simulink model "Starfighter_6DoF_runsim_waypoint"  (R2013b)
settings: Solver=ode4  StartTime=0.0  StopTime=1  FixedStep=.01  MaxStep=.004  RelTol=1e-5
values from neighbouring files (symbols this model uses):
  a = 967.78    [LocusTrans.m]    (also in runsim_Starfighter_6DoF_Waypoint.m)
  ac = [0 0 0]    [LocusTrans.m]    (also in runsim_Starfighter_6DoF_Waypoint.m)
  b = 21.9    [LocusTrans.m]    (also in runsim_Starfighter_6DoF_Waypoint.m)
  cbar = 9.6    [LocusTrans.m]    (also in runsim_Starfighter_6DoF_Waypoint.m)
  cda = 0.384    [LocusTrans.m]    (also in runsim_Starfighter_6DoF_Waypoint.m)
  cdde = 0    [LocusTrans.m]    (also in runsim_Starfighter_6DoF_Waypoint.m)
  cdo = 0.048    [LocusTrans.m]    (also in runsim_Starfighter_6DoF_Waypoint.m)
  cg = [0 0 0]    [LocusTrans.m]    (also in runsim_Starfighter_6DoF_Waypoint.m)
  cla = 2.005    [LocusTrans.m]    (also in runsim_Starfighter_6DoF_Waypoint.m)
  cladot = 0.82    [LocusTrans.m]    (also in runsim_Starfighter_6DoF_Waypoint.m)
  clb = -0.093    [LocusTrans.m]    (also in runsim_Starfighter_6DoF_Waypoint.m)
  clda = 0.0173    [LocusTrans.m]    (also in runsim_Starfighter_6DoF_Waypoint.m)
  clde = 0.523    [LocusTrans.m]    (also in runsim_Starfighter_6DoF_Waypoint.m)
  cldr = 0.0079    [LocusTrans.m]    (also in runsim_Starfighter_6DoF_Waypoint.m)
  clo = 0.122    [LocusTrans.m]    (also in runsim_Starfighter_6DoF_Waypoint.m)
  clp = -0.272    [LocusTrans.m]    (also in runsim_Starfighter_6DoF_Waypoint.m)
  clq = 1.9    [LocusTrans.m]    (also in runsim_Starfighter_6DoF_Waypoint.m)
  clr = 0.154    [LocusTrans.m]    (also in runsim_Starfighter_6DoF_Waypoint.m)
  cma = -1.308    [LocusTrans.m]    (also in runsim_Starfighter_6DoF_Waypoint.m)
  cmadot = -2.05    [LocusTrans.m]    (also in runsim_Starfighter_6DoF_Waypoint.m)
  cmde = -1.31    [LocusTrans.m]    (also in runsim_Starfighter_6DoF_Waypoint.m)
  cmo = -0.028    [LocusTrans.m]    (also in runsim_Starfighter_6DoF_Waypoint.m)
  cmq = -4.83    [LocusTrans.m]    (also in runsim_Starfighter_6DoF_Waypoint.m)
  cnb = 0.242    [LocusTrans.m]    (also in runsim_Starfighter_6DoF_Waypoint.m)
  cnda = -0.0025    [LocusTrans.m]    (also in runsim_Starfighter_6DoF_Waypoint.m)
  cndr = -0.0435    [LocusTrans.m]    (also in runsim_Starfighter_6DoF_Waypoint.m)
  cnp = -0.093    [LocusTrans.m]    (also in runsim_Starfighter_6DoF_Waypoint.m)
  cnr = -0.649    [LocusTrans.m]    (also in runsim_Starfighter_6DoF_Waypoint.m)
  cyb = -1.045    [LocusTrans.m]    (also in runsim_Starfighter_6DoF_Waypoint.m)
  cyda = 0    [LocusTrans.m]    (also in runsim_Starfighter_6DoF_Waypoint.m)
  cydr = 0.087    [LocusTrans.m]    (also in runsim_Starfighter_6DoF_Waypoint.m)
  cyp = 0    [LocusTrans.m]    (also in runsim_Starfighter_6DoF_Waypoint.m)
  cyr = 0    [LocusTrans.m]    (also in runsim_Starfighter_6DoF_Waypoint.m)
  de0 = -4.1938979*pi/180    (= -0.0731973268475)    [LocusTrans.m]    (also in runsim_Starfighter_6DoF_Waypoint.m)
  dT0 = 5795.5876705721688901230688059874    (= 5795.58767057)    [LocusTrans.m]    (also in runsim_Starfighter_6DoF_Waypoint.m = 0.4868)
  eng = [0 0 0]    [LocusTrans.m]    (also in runsim_Starfighter_6DoF_Waypoint.m)
  inialt = 55000    [runsim_Starfighter_6DoF_Waypoint.m]
  initalt = 0    [LocusTrans.m]    (also in runsim_Starfighter_6DoF_Waypoint.m = 55000)
  initeast = 0    [LocusTrans.m]    (also in runsim_Starfighter_6DoF_Waypoint.m)
  initnorth = 0    [LocusTrans.m]    (also in runsim_Starfighter_6DoF_Waypoint.m)
  initp = p0    (= 0)    [LocusTrans.m]    (also in runsim_Starfighter_6DoF_Waypoint.m)
  initpitch = theta0    (= 0.0519025210107)    [LocusTrans.m]    (also in runsim_Starfighter_6DoF_Waypoint.m)
  initq = q0    (= 0)    [LocusTrans.m]    (also in runsim_Starfighter_6DoF_Waypoint.m)
  initr = r0    (= 0)    [LocusTrans.m]    (also in runsim_Starfighter_6DoF_Waypoint.m)
  initroll = phi0    (= 0)    [LocusTrans.m]    (also in runsim_Starfighter_6DoF_Waypoint.m)
  initu = u0    [LocusTrans.m]    (also in runsim_Starfighter_6DoF_Waypoint.m)
  initv = v0    [LocusTrans.m]    (also in runsim_Starfighter_6DoF_Waypoint.m)
  initw = w0    [LocusTrans.m]    (also in runsim_Starfighter_6DoF_Waypoint.m)
  inityaw = 0.0    (= 0)    [LocusTrans.m]    (also in runsim_Starfighter_6DoF_Waypoint.m)
  Ix = 3600    [LocusTrans.m]    (also in runsim_Starfighter_6DoF_Waypoint.m)
  Ixz = 0    [LocusTrans.m]    (also in runsim_Starfighter_6DoF_Waypoint.m)
  Iy = 59000    [LocusTrans.m]    (also in runsim_Starfighter_6DoF_Waypoint.m)
  Iz = 60000    [LocusTrans.m]    (also in runsim_Starfighter_6DoF_Waypoint.m)
  K_phi = 10    [runsim_Starfighter_6DoF_Waypoint.m]
  rho = .002378*(1-.0000068756*     h)^4.2561    (= 0.000314842619782)    [LocusTrans.m]    (also in runsim_Starfighter_6DoF_Waypoint.m)
  sw = 196    [LocusTrans.m]    (also in runsim_Starfighter_6DoF_Waypoint.m)
  T_max = 11905    [runsim_Starfighter_6DoF_Waypoint.m]
  u0 = Vt0*cos(alpha0)*cos(beta0)    [LocusTrans.m]    (also in runsim_Starfighter_6DoF_Waypoint.m)
  Vt0 = 1742    [Control.m]    (also in LocusTrans.m; runsim_Starfighter_6DoF_Waypoint.m)
  weight = 16300    [runsim_Starfighter_6DoF_Waypoint.m]
  Xw = (1/u0)*Xa    [LocusTrans.m]    (also in runsim_Starfighter_6DoF_Waypoint.m = 2*[52*Vt0, 104*Vt0, 104*Vt0, 52*Vt0, 0])
libraries: simulink x6, dspswit3 x1
(part 1 of 2)
settings Model: ExtModeAutoUpdateStatusClock=off  Creator=andersop  LastModifiedBy=mittalk1
settings SolverCC: InitialStep=.004
settings DataIOCC: SignalLoggingSaveFormat=ModelDataLogs  SaveState=on  SignalLoggingName=sigsOut
settings OptimizationCC: ExpressionDepthLimit=2147483647  InitFltsAndDblsToZero=on
settings DebuggingCC: SaveWithParameterizedLinksMsg=none  SignalResolutionControl=TryResolveAllWithWarning  SolverPrmCheckMsg=none  MultiTaskDSMMsg=warning  MultiTaskCondExecSysMsg=none  FcnCallInpInsideContextMsg=UseLocalSettings  StateNameClashWarn=warning
settings HardwareCC: TargetUnknown=on
settings RTWCC: IncludeERTFirstTime=on
settings GRTTargetCC: TargetFcnLib=ansi_tfl_tmw.mat  ModelReferenceCompliant=off  CombineOutputUpdateFcns=off  MatFileLogging=off  GRTInterface=on

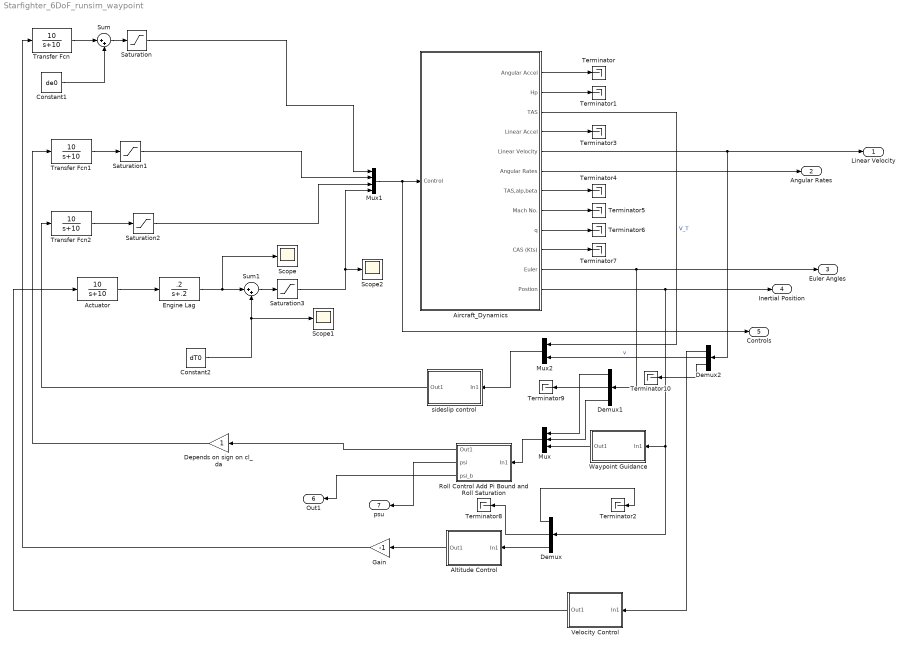
== system Starfighter_6DoF_runsim_waypoint ==
  Actuator : TransferFcn  Numerator=[10]  Denominator=[1 10]
  Aircraft_Dynamics : Subsystem
  Altitude Control : Subsystem
  Constant1 : Constant  Value=de0
  Constant2 : Constant  Value=dT0
  Demux : Demux  Outputs=3
  Demux1 : Demux  Outputs=3
  Demux2 : Demux  Outputs=3
  Depends on sign on cl_da : Gain
  Engine Lag : TransferFcn  Numerator=[.2]  Denominator=[1 .2]
  Gain : Gain  Gain=-1
  Mux : Mux  Inputs=3
  Mux1 : Mux
  Mux2 : Mux  Inputs=2
  Roll Control Add Pi Bound and Roll Saturation : Subsystem
  Saturation : Saturate  UpperLimit=30*pi/180  LowerLimit=-30*pi/180
  Saturation1 : Saturate  UpperLimit=40*pi/180  LowerLimit=-40*pi/180
  Saturation2 : Saturate  UpperLimit=30*pi/180  LowerLimit=-30*pi/180
  Saturation3 : Saturate  UpperLimit=1  LowerLimit=0
  Scope : Scope
      settings: YMin=0  YMax=0.025
  Scope1 : Scope
      settings: YMin=0.4868  YMax=0.4868
  Scope2 : Scope
      settings: YMin=0.485  YMax=0.5125  SaveName=ScopeData2
  Sum : Sum  Inputs=|++
  Sum1 : Sum  Inputs=|++
  Terminator{,1..10} (11 alike) : Terminator
  Transfer Fcn : TransferFcn  Numerator=[10]  Denominator=[1 10]
  Transfer Fcn1 : TransferFcn  Numerator=[10]  Denominator=[1 10]
  Transfer Fcn2 : TransferFcn  Numerator=[10]  Denominator=[1 10]
  Velocity Control : Subsystem
  Waypoint Guidance : Subsystem
  sideslip control : Subsystem
  Linear Velocity : Outport
  Angular Rates : Outport  Port=2
  Euler Angles : Outport  Port=3
  Inertial Position : Outport  Port=4
  Controls : Outport  Port=5
  Out1 : Outport  Port=6
  psu : Outport  Port=7
  wires:
  Aircraft_Dynamics/11(Euler) -> Demux1/1, Euler Angles/1
  Saturation3/1 -> Scope2/1, Mux1/4
  Mux1/1 -> Aircraft_Dynamics/1(Control), Controls/1
  Saturation/1 -> Mux1/1
  Aircraft_Dynamics/6(Angular Rates) -> Angular Rates/1
  Aircraft_Dynamics/5(Linear Velocity) -> Demux2/1, Linear Velocity/1
  Saturation2/1 -> Mux1/3
  Saturation1/1 -> Mux1/2
  Aircraft_Dynamics/1(Angular Accel) -> Terminator/1
  Aircraft_Dynamics/2(Hp) -> Terminator1/1
  Aircraft_Dynamics/3(TAS) -> Mux2/1  "V_T"
  Aircraft_Dynamics/4(Linear Accel) -> Terminator3/1
  Aircraft_Dynamics/7(TAS,alp,beta) -> Terminator4/1
  Aircraft_Dynamics/8(Mach No.) -> Terminator5/1
  Aircraft_Dynamics/10(CAS (Kts)) -> Terminator7/1
  Aircraft_Dynamics/9(q) -> Terminator6/1
  Sum/1 -> Saturation/1
  Constant1/1 -> Sum/2
  Transfer Fcn/1 -> Sum/1
  Transfer Fcn1/1 -> Saturation1/1
  Aircraft_Dynamics/12(Postion) -> Demux/1, Waypoint Guidance/1(In1), Inertial Position/1
  Waypoint Guidance/1(Out1) -> Mux/3
  Demux1/1 -> Mux/1
  Demux1/3 -> Mux/2
  Mux/1 -> Roll Control Add Pi Bound and Roll Saturation/1(In1)
  Depends on sign on cl_da/1 -> Transfer Fcn1/1
  Gain/1 -> Transfer Fcn/1
  Demux/3 -> Altitude Control/1(In1)
  Altitude Control/1(Out1) -> Gain/1
  Demux2/2 -> Mux2/2  "v"
  Transfer Fcn2/1 -> Saturation2/1
  sideslip control/1(Out1) -> Transfer Fcn2/1
  Demux/1 -> Terminator2/1
  Demux/2 -> Terminator8/1
  Demux1/2 -> Terminator9/1
  Demux2/1 -> Velocity Control/1(In1)
  Constant2/1 -> Scope1/1, Sum1/2
  Engine Lag/1 -> Scope/1, Sum1/1
  Actuator/1 -> Engine Lag/1
  Sum1/1 -> Saturation3/1
  Velocity Control/1(Out1) -> Actuator/1
  Demux2/3 -> Terminator10/1
  Roll Control Add Pi Bound and Roll Saturation/2(psi) -> psu/1
  Roll Control Add Pi Bound and Roll Saturation/3(psi_b) -> Out1/1
  Mux2/1 -> sideslip control/1(In1)
  Roll Control Add Pi Bound and Roll Saturation/1(Out1) -> Depends on sign on cl_da/1

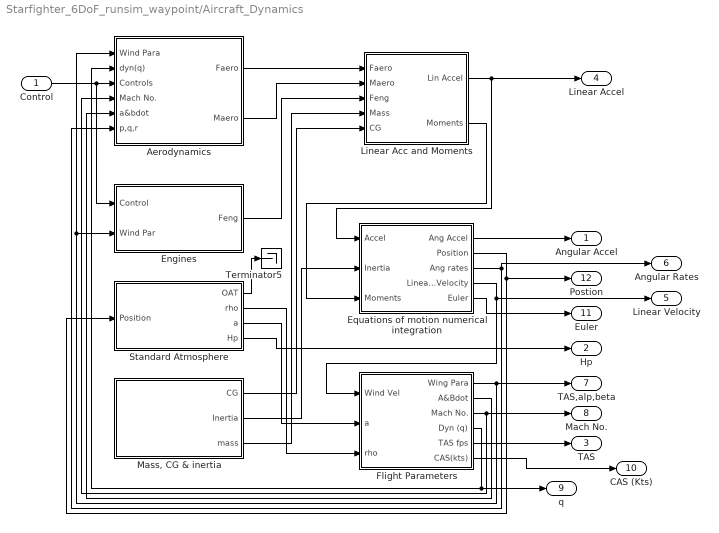
== system Starfighter_6DoF_runsim_waypoint/Aircraft_Dynamics ==
  Control : Inport
  Aerodynamics : Subsystem
  Engines : Subsystem
  "Equations of motion numerical integration " : Subsystem
  Flight Parameters : Subsystem
  Linear Acc and Moments : Subsystem
  "Mass, CG & inertia" : Subsystem
  Standard Atmosphere : Subsystem
  Terminator5 : Terminator
  Angular Accel : Outport
  Hp : Outport  Port=2
  TAS : Outport  Port=3
  Linear Accel : Outport  Port=4
  Linear Velocity : Outport  Port=5
  Angular Rates : Outport  Port=6
  TAS,alp,beta : Outport  Port=7
  Mach No. : Outport  Port=8
  q : Outport  Port=9
  CAS (Kts) : Outport  Port=10
  Euler : Outport  Port=11
  Postion : Outport  Port=12
  wires:
  Aerodynamics/1(Faero) -> Linear Acc and Moments/1(Faero)
  Aerodynamics/2(Maero) -> Linear Acc and Moments/2(Maero)
  Control/1 -> Aerodynamics/3(Controls), Engines/1(Control)
  Engines/1(Feng) -> Linear Acc and Moments/3(Feng)
  "Mass, CG & inertia"/1(CG) -> Linear Acc and Moments/5(CG)
  "Mass, CG & inertia"/2(Inertia) -> "Equations of motion numerical integration "/2(Inertia)
  Linear Acc and Moments/1(Lin Accel) -> "Equations of motion numerical integration "/1(Accel), Linear Accel/1
  Linear Acc and Moments/2(Moments) -> "Equations of motion numerical integration "/3(Moments)
  "Equations of motion numerical integration "/3(Ang rates) -> Aerodynamics/6(p,q,r), Angular Rates/1
  "Equations of motion numerical integration "/4(Linear Velocity) -> Flight Parameters/1(Wind Vel), Linear Velocity/1
  Flight Parameters/1(Wing Para) -> TAS,alp,beta/1, Aerodynamics/1(Wind Para), Engines/2(Wind Par)
  Flight Parameters/4(Dyn (q)) -> Aerodynamics/2(dyn(q)), q/1
  Flight Parameters/3(Mach No.) -> Mach No./1, Aerodynamics/4(Mach No.)
  Flight Parameters/2(A&Bdot) -> Aerodynamics/5(a&bdot)
  "Equations of motion numerical integration "/2(Position) -> Postion/1, Standard Atmosphere/1(Position)
  "Equations of motion numerical integration "/1(Ang Accel) -> Angular Accel/1
  Standard Atmosphere/4(Hp) -> Hp/1
  Flight Parameters/5(TAS fps) -> TAS/1
  Flight Parameters/6(CAS(kts)) -> CAS (Kts)/1
  "Equations of motion numerical integration "/5(Euler) -> Euler/1
  Standard Atmosphere/3(a) -> Flight Parameters/2(a)
  Standard Atmosphere/2(rho) -> Flight Parameters/3(rho)
  "Mass, CG & inertia"/3(mass) -> Linear Acc and Moments/4(Mass)
  Standard Atmosphere/1(OAT) -> Terminator5/1

== system Starfighter_6DoF_runsim_waypoint/Altitude Control ==
  In1 : Inport
  Altitude PID Controller : simulink/Continuous/PID Controller  Controller=PID  TimeDomain=Continuous-time  SampleTime=1  IntegratorMethod=Forward Euler  FilterMethod=Forward Euler  Form=Parallel  P=5.28484698542776e-05  I=1.87875420337088e-07  D=0.00194166371372168  N=0.684337429388764  InitialConditionSource=internal  InitialConditionForIntegrator=0  InitialConditionForFilter=0  ExternalReset=none  LimitOutput=off  UpperSaturationLimit=inf  LowerSaturationLimit=-inf  LinearizeAsGain=on  AntiWindupMode=none  Kb=1  TrackingMode=off  Kt=1  PParamMin=[]  PParamMax=[]  IParamMin=[]  IParamMax=[]  DParamMin=[]  DParamMax=[]  NParamMin=[]  NParamMax=[]  KbParamMin=[]  KbParamMax=[]  KtParamMin=[]  KtParamMax=[]  POutMin=[]  POutMax=[]  IOutMin=[]  IOutMax=[]  DOutMin=[]  DOutMax=[]  NOutMin=[]  NOutMax=[]  KbOutMin=[]  KbOutMax=[]  KtOutMin=[]  KtOutMax=[]  IntegratorOutMin=[]  IntegratorOutMax=[]  FilterOutMin=[]  FilterOutMax=[]  SumOutMin=[]  SumOutMax=[]  SumI1OutMin=[]  SumI1OutMax=[]  SumI2OutMin=[]  SumI2OutMax=[]  SumI3OutMin=[]  SumI3OutMax=[]  SumDOutMin=[]  SumDOutMax=[]  SaturationOutMin=[]  SaturationOutMax=[]  IntegratorContinuousStateAttributes=''  IntegratorStateMustResolveToSignalObject=off  IntegratorRTWStateStorageClass=Auto  FilterContinuousStateAttributes=''  FilterStateMustResolveToSignalObject=off  FilterRTWStateStorageClass=Auto
  Constant : Constant  Value=inialt
  Sum1 : Sum  Inputs=|-+
  Out1 : Outport
  wires:
  Sum1/1 -> Altitude PID Controller/1
  In1/1 -> Sum1/1
  Altitude PID Controller/1 -> Out1/1
  Constant/1 -> Sum1/2

== system Starfighter_6DoF_runsim_waypoint/Roll Control Add Pi Bound and Roll Saturation ==
  In1 : Inport
  Demux : Demux  Outputs=3
  Gain : Gain  Gain=K_phi
  PID Controller : simulink/Continuous/PID Controller  Controller=PID  TimeDomain=Continuous-time  SampleTime=1  IntegratorMethod=Forward Euler  FilterMethod=Forward Euler  Form=Parallel  P=0.0237928230779275  I=0.000453455739705604  D=0.0522613184684565  N=1.14124341327547  InitialConditionSource=internal  InitialConditionForIntegrator=0  InitialConditionForFilter=0  ExternalReset=none  LimitOutput=off  UpperSaturationLimit=inf  LowerSaturationLimit=-inf  LinearizeAsGain=on  AntiWindupMode=none  Kb=1  TrackingMode=off  Kt=1  PParamMin=[]  PParamMax=[]  IParamMin=[]  IParamMax=[]  DParamMin=[]  DParamMax=[]  NParamMin=[]  NParamMax=[]  KbParamMin=[]  KbParamMax=[]  KtParamMin=[]  KtParamMax=[]  POutMin=[]  POutMax=[]  IOutMin=[]  IOutMax=[]  DOutMin=[]  DOutMax=[]  NOutMin=[]  NOutMax=[]  KbOutMin=[]  KbOutMax=[]  KtOutMin=[]  KtOutMax=[]  IntegratorOutMin=[]  IntegratorOutMax=[]  FilterOutMin=[]  FilterOutMax=[]  SumOutMin=[]  SumOutMax=[]  SumI1OutMin=[]  SumI1OutMax=[]  SumI2OutMin=[]  SumI2OutMax=[]  SumI3OutMin=[]  SumI3OutMax=[]  SumDOutMin=[]  SumDOutMax=[]  SaturationOutMin=[]  SaturationOutMax=[]  IntegratorContinuousStateAttributes=''  IntegratorStateMustResolveToSignalObject=off  IntegratorRTWStateStorageClass=Auto  FilterContinuousStateAttributes=''  FilterStateMustResolveToSignalObject=off  FilterRTWStateStorageClass=Auto
  Saturation : Saturate  UpperLimit=40*(pi/180)  LowerLimit=-40*(pi/180)
  Sum : Sum  Inputs=|-+
  Sum1 : Sum  Inputs=|-+
  pi Bound1 : Subsystem  mask(pi bound){}
      mask help: Bounds the input angle to [-pi, pi]. When -pi bound is exceeded the output wraps back to pi; when the pi bound is exceeded the output wraps back to -pi.
      mask Help:
      | Bounds the input angle to [-pi, pi]. When -pi bound is exceeded the output wraps back to pi; when the pi bound is exceeded the output wraps back to -pi.
      | <P><B>Input:</B> any angle in radians, from -Inf to Inf;</P>
      | <P><B>Output:</B> an angle in radians between -pi and pi.</P>
  Out1 : Outport
  psi : Outport  Port=2
  psi_b : Outport  Port=3
  wires:
  In1/1 -> Demux/1
  Demux/1 -> Sum1/1  "phi (roll)"
  Demux/2 -> psi/1, Sum/1  "psi (yaw)"
  Demux/3 -> Sum/2, psi_b/1  "psi_b (bearing)"
  Sum1/1 -> PID Controller/1
  Saturation/1 -> Sum1/2
  Gain/1 -> Saturation/1
  PID Controller/1 -> Out1/1  "psi_b (bearing)"
  Sum/1 -> pi Bound1/1(In)  "dpsi_com"
  pi Bound1/1(Out) -> Gain/1

== system Starfighter_6DoF_runsim_waypoint/Velocity Control ==
  In1 : Inport
  Altitude PID Controller : simulink/Continuous/PID Controller  Controller=PID  TimeDomain=Continuous-time  SampleTime=1  IntegratorMethod=Forward Euler  FilterMethod=Forward Euler  Form=Parallel  P=6.68504925199233e-05  I=6.07478695378791e-07  D=0  N=100  InitialConditionSource=internal  InitialConditionForIntegrator=0  InitialConditionForFilter=0  ExternalReset=none  LimitOutput=off  UpperSaturationLimit=inf  LowerSaturationLimit=-inf  LinearizeAsGain=on  AntiWindupMode=none  Kb=1  TrackingMode=off  Kt=1  PParamMin=[]  PParamMax=[]  IParamMin=[]  IParamMax=[]  DParamMin=[]  DParamMax=[]  NParamMin=[]  NParamMax=[]  KbParamMin=[]  KbParamMax=[]  KtParamMin=[]  KtParamMax=[]  POutMin=[]  POutMax=[]  IOutMin=[]  IOutMax=[]  DOutMin=[]  DOutMax=[]  NOutMin=[]  NOutMax=[]  KbOutMin=[]  KbOutMax=[]  KtOutMin=[]  KtOutMax=[]  IntegratorOutMin=[]  IntegratorOutMax=[]  FilterOutMin=[]  FilterOutMax=[]  SumOutMin=[]  SumOutMax=[]  SumI1OutMin=[]  SumI1OutMax=[]  SumI2OutMin=[]  SumI2OutMax=[]  SumI3OutMin=[]  SumI3OutMax=[]  SumDOutMin=[]  SumDOutMax=[]  SaturationOutMin=[]  SaturationOutMax=[]  IntegratorContinuousStateAttributes=''  IntegratorStateMustResolveToSignalObject=off  IntegratorRTWStateStorageClass=Auto  FilterContinuousStateAttributes=''  FilterStateMustResolveToSignalObject=off  FilterRTWStateStorageClass=Auto
  Constant : Constant  Value=u0
  Sum1 : Sum  Inputs=|-+
  Out1 : Outport
  wires:
  Sum1/1 -> Altitude PID Controller/1
  In1/1 -> Sum1/1
  Altitude PID Controller/1 -> Out1/1
  Constant/1 -> Sum1/2

== system Starfighter_6DoF_runsim_waypoint/Waypoint Guidance ==
  In1 : Inport
  Compare To Constant : simulink/Logic and Bit Operations/Compare To Constant  relop=<=  const=3*Vt0  OutDataTypeStr=boolean
  Compare To Constant1 : simulink/Logic and Bit Operations/Compare To Constant  relop=>  const=length(Xw)  OutDataTypeStr=boolean
  Counter : dspswit3/Counter  Direction=Up  CountEvent=Rising edge  CounterSize=User defined  MaxCount=6  InitialCount=1  Output=Count and Hit  HitValue=32  ResetInput=on  SamplesPerFrame=1  Ts=1  CntDtype=double  HitDtype=Logical
  Demux1 : Demux  Outputs=3
  MATLAB Function : MATLAB Function  TreatAsAtomicUnit=on
  Memory : Memory  X0=1
  Stop Simulation : Stop
  Terminator : Terminator
  Out1 : Outport
  wires:
  In1/1 -> Demux1/1
  Compare To Constant/1 -> Counter/1
  Counter/1 -> Memory/1
  Compare To Constant1/1 -> Stop Simulation/1
  Demux1/1 -> MATLAB Function/1(X)
  Demux1/3 -> MATLAB Function/3(Z)
  Demux1/2 -> MATLAB Function/2(Y)
  MATLAB Function/2(psi_b) -> Out1/1
  Memory/1 -> MATLAB Function/4(count), Compare To Constant1/1
  MATLAB Function/1(d) -> Compare To Constant/1
  Counter/2 -> Terminator/1

== system Starfighter_6DoF_runsim_waypoint/sideslip control ==
  note: V_T
  In1 : Inport
  Altitude PID Controller : simulink/Continuous/PID Controller  Controller=PID  TimeDomain=Continuous-time  SampleTime=1  IntegratorMethod=Forward Euler  FilterMethod=Forward Euler  Form=Parallel  P=0  I=0.130392267161925  D=0  N=100  InitialConditionSource=internal  InitialConditionForIntegrator=0  InitialConditionForFilter=0  ExternalReset=none  LimitOutput=off  UpperSaturationLimit=inf  LowerSaturationLimit=-inf  LinearizeAsGain=on  AntiWindupMode=none  Kb=1  TrackingMode=off  Kt=1  PParamMin=[]  PParamMax=[]  IParamMin=[]  IParamMax=[]  DParamMin=[]  DParamMax=[]  NParamMin=[]  NParamMax=[]  KbParamMin=[]  KbParamMax=[]  KtParamMin=[]  KtParamMax=[]  POutMin=[]  POutMax=[]  IOutMin=[]  IOutMax=[]  DOutMin=[]  DOutMax=[]  NOutMin=[]  NOutMax=[]  KbOutMin=[]  KbOutMax=[]  KtOutMin=[]  KtOutMax=[]  IntegratorOutMin=[]  IntegratorOutMax=[]  FilterOutMin=[]  FilterOutMax=[]  SumOutMin=[]  SumOutMax=[]  SumI1OutMin=[]  SumI1OutMax=[]  SumI2OutMin=[]  SumI2OutMax=[]  SumI3OutMin=[]  SumI3OutMax=[]  SumDOutMin=[]  SumDOutMax=[]  SaturationOutMin=[]  SaturationOutMax=[]  IntegratorContinuousStateAttributes=''  IntegratorStateMustResolveToSignalObject=off  IntegratorRTWStateStorageClass=Auto  FilterContinuousStateAttributes=''  FilterStateMustResolveToSignalObject=off  FilterRTWStateStorageClass=Auto
  Constant : Constant  Value=0
  Demux : Demux  Outputs=2
  Divide : Product  Inputs=/*
  Sum1 : Sum  Inputs=|-+
  Trigonometric Function : Trigonometry  Operator=asin
  Out1 : Outport
  wires:
  Sum1/1 -> Altitude PID Controller/1
  Altitude PID Controller/1 -> Out1/1
  Constant/1 -> Sum1/2
  In1/1 -> Demux/1
  Trigonometric Function/1 -> Sum1/1
  Demux/2 -> Divide/2  "v"
  Divide/1 -> Trigonometric Function/1
  Demux/1 -> Divide/1

== system Starfighter_6DoF_runsim_waypoint/Aircraft_Dynamics/Aerodynamics ==
  Wind Para : Inport
  dyn(q) : Inport  Port=2
  Controls : Inport  Port=3
  Mach No. : Inport  Port=4
  a&bdot : Inport  Port=5
  p,q,r : Inport  Port=6
  Aero Forces and Moments : Subsystem
  CD : Subsystem
  CL : Subsystem
  CM : Subsystem
  CN : Subsystem
  CY : Subsystem
  Croll : Subsystem
  Faero : Outport
  Maero : Outport  Port=2
  wires:
  Wind Para/1 -> CL/1(Wind Parameters), CY/1(Wind Parameters), Aero Forces and Moments/5(Wind Para), CN/1(Wind Parameters), Croll/1(Wind Parameters), CM/1(Wind Parameters), CD/1(Wind Parameters)
  CL/1(CL) -> Aero Forces and Moments/4(CL)
  Mach No./1 -> CM/3(Mach No.), CN/3(Mach No.), Croll/3(Mach No.), CY/3(Mach No.), CL/3(Mach No.), CD/3(Mach No.)
  a&bdot/1 -> CL/4(a&bdot), CM/4(a&bdot)
  p,q,r/1 -> CM/5(P,q,r), CN/4(P,q,r), Croll/4(P,q,r), CY/4(P,q,r), CL/5(P,q,r)
  Controls/1 -> CM/2(Controls), CD/2(Controls), CN/2(Controls), Croll/2(Controls), CY/2(Controls), CL/2(Controls)
  CD/1(CD) -> Aero Forces and Moments/2(CD)
  CN/1(CN) -> Aero Forces and Moments/8(CN)
  Croll/1(Croll) -> Aero Forces and Moments/6(Croll)
  CY/1(CY) -> Aero Forces and Moments/3(CY)
  CM/1(CM) -> Aero Forces and Moments/7(CM)
  dyn(q)/1 -> Aero Forces and Moments/1(dyn(q))
  Aero Forces and Moments/1(Faero) -> Faero/1
  Aero Forces and Moments/2(Maero) -> Maero/1

== system Starfighter_6DoF_runsim_waypoint/Aircraft_Dynamics/Engines ==
  Control : Inport
  Wind Par : Inport  Port=2
  Demux : Demux
  Demux1 : Demux  Outputs=3
  Display : Display
  Max Power : Constant  Value=T_max
  Product : Product  RndMeth=Zero
  Terminator{,1..5} (6 alike) : Terminator
  Feng : Outport
  wires:
  Max Power/1 -> Product/2
  Control/1 -> Demux/1
  Demux/4 -> Product/1
  Demux/1 -> Terminator/1
  Demux/2 -> Terminator1/1
  Demux/3 -> Terminator2/1
  Product/1 -> Feng/1, Display/1
  Wind Par/1 -> Demux1/1
  Demux1/1 -> Terminator5/1
  Demux1/2 -> Terminator4/1
  Demux1/3 -> Terminator3/1

== system Starfighter_6DoF_runsim_waypoint/Aircraft_Dynamics/Equations of motion numerical integration  ==
  Accel : Inport
  Inertia : Inport  Port=2
  Moments : Inport  Port=3
  Flat Earth Navigation : Subsystem
  Force Equations : Subsystem
  Gravity Model : Subsystem
  Inert-body : Subsystem
  Kinematic Equiations : Subsystem
  Moment Equations : Subsystem
  Ang Accel : Outport
  Position : Outport  Port=2
  Ang rates : Outport  Port=3
  Linear Velocity : Outport  Port=4
  Euler : Outport  Port=5
  wires:
  Moment Equations/1(Ang Rates) -> Kinematic Equiations/1(Rates), Force Equations/3(Rates), Ang rates/1
  Kinematic Equiations/1(Euler angles) -> Flat Earth Navigation/1(Euler Angles), Inert-body/1(Euler), Euler/1
  Force Equations/1(Lin Vel) -> Linear Velocity/1, Flat Earth Navigation/2(Velocity)
  Accel/1 -> Force Equations/1(Accel)
  Inertia/1 -> Moment Equations/1(Inertia)
  Gravity Model/1(Gravity) -> Force Equations/2(Gravity)
  Moments/1 -> Moment Equations/2(Moments)
  Moment Equations/2(Ang Accel) -> Ang Accel/1
  Flat Earth Navigation/1(Position) -> Position/1
  Inert-body/1(NEDtoBC) -> Force Equations/4(NEDtoABC)

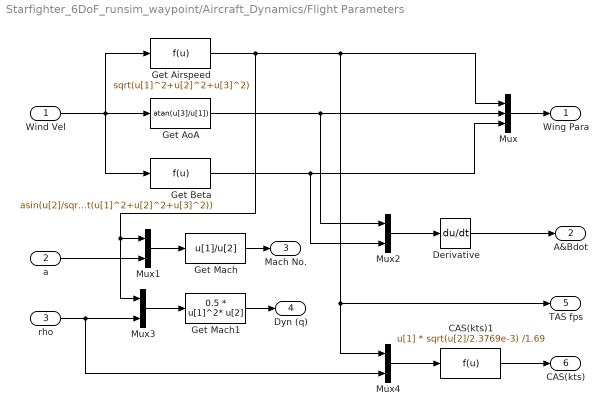
== system Starfighter_6DoF_runsim_waypoint/Aircraft_Dynamics/Flight Parameters ==
  Wind Vel : Inport
  a : Inport  Port=2
  rho : Inport  Port=3
  CAS(kts)1 : Fcn  Expr=u[1] * sqrt(u[2]/2.3769e-3) /1.69
  Derivative : Derivative
  Get Airspeed : Fcn  Expr=sqrt(u[1]^2+u[2]^2+u[3]^2)
  Get AoA : Fcn  Expr=atan(u[3]/u[1])
  Get Beta : Fcn  Expr=asin(u[2]/sqrt(u[1]^2+u[2]^2+u[3]^2))
  Get Mach : Fcn  Expr=u[1]/u[2]
  Get Mach1 : Fcn  Expr=0.5 * u[1]^2* u[2]
  Mux : Mux  Inputs=3
  Mux{1..4} (4 alike) : Mux  Inputs=2
  Wing Para : Outport
  A&Bdot : Outport  Port=2
  Mach No. : Outport  Port=3
  Dyn (q) : Outport  Port=4
  TAS fps : Outport  Port=5
  CAS(kts) : Outport  Port=6
  wires:
  Wind Vel/1 -> Get AoA/1, Get Airspeed/1, Get Beta/1
  Get AoA/1 -> Mux/2, Mux2/1
  Get Airspeed/1 -> Mux1/1, Mux3/1, TAS fps/1, Mux4/1, Mux/1
  Get Beta/1 -> Mux/3, Mux2/2
  Mux/1 -> Wing Para/1
  Mux1/1 -> Get Mach/1
  a/1 -> Mux1/2
  Mux2/1 -> Derivative/1
  Derivative/1 -> A&Bdot/1
  Get Mach/1 -> Mach No./1
  rho/1 -> Mux3/2, Mux4/2
  Mux3/1 -> Get Mach1/1
  Get Mach1/1 -> Dyn (q)/1
  Mux4/1 -> CAS(kts)1/1
  CAS(kts)1/1 -> CAS(kts)/1

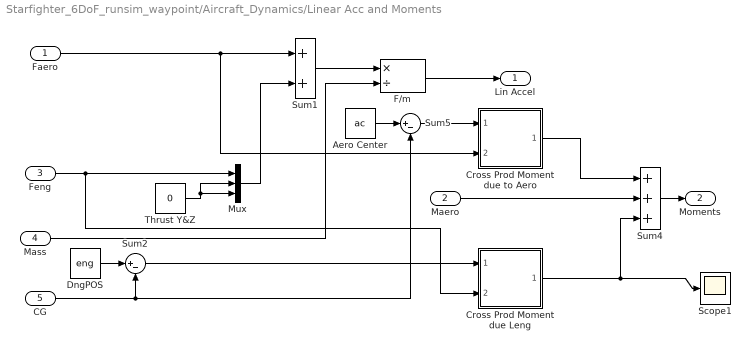
== system Starfighter_6DoF_runsim_waypoint/Aircraft_Dynamics/Linear Acc and Moments ==
  Faero : Inport
  Maero : Inport  Port=2
  Feng : Inport  Port=3
  Mass : Inport  Port=4
  CG : Inport  Port=5
  Aero Center : Constant  Value=ac
  Cross Prod Moment due Leng : Subsystem
  Cross Prod Moment due to Aero : Subsystem
  DngPOS : Constant  Value=eng
  F/m : Product  Inputs=*/  SaturateOnIntegerOverflow=on  OutDataTypeStr=Inherit: Same as first input
  Mux : Mux  Inputs=3
  Scope1 : Scope
      settings: YMin=-0.2  YMax=0.8  SaveName=ScopeData3
  Sum1 : Sum  SaturateOnIntegerOverflow=on
  Sum2 : Sum  Inputs=|+-  SaturateOnIntegerOverflow=on
  Sum4 : Sum  Inputs=+++  SaturateOnIntegerOverflow=on
  Sum5 : Sum  Inputs=|+-  SaturateOnIntegerOverflow=on
  Thrust Y&Z : Constant  Value=0
  Lin Accel : Outport
  Moments : Outport  Port=2
  wires:
  Feng/1 -> Cross Prod Moment due Leng/2(Vec 2), Mux/1
  Thrust Y&Z/1 -> Mux/2, Mux/3
  Faero/1 -> Sum1/1, Cross Prod Moment due to Aero/2(Vec 2)
  Mux/1 -> Sum1/2
  Sum1/1 -> F/m/1
  Mass/1 -> F/m/2
  F/m/1 -> Lin Accel/1
  CG/1 -> Sum2/2, Sum5/2
  Aero Center/1 -> Sum5/1
  Sum5/1 -> Cross Prod Moment due to Aero/1(Vec 1)
  Maero/1 -> Sum4/2
  Sum4/1 -> Moments/1
  Cross Prod Moment due to Aero/1(X Prod) -> Sum4/1
  Sum2/1 -> Cross Prod Moment due Leng/1(Vec 1)
  Cross Prod Moment due Leng/1(X Prod) -> Sum4/3, Scope1/1
  DngPOS/1 -> Sum2/1

== system Starfighter_6DoF_runsim_waypoint/Aircraft_Dynamics/Mass, CG & inertia ==
  Mux1 : Mux
  cg : Constant  Value=cg
  jx : Constant  Value=Ix
  jxz : Constant  Value=Ixz
  jy : Constant  Value=Iy
  jz : Constant  Value=Iz
  mass2 : Constant  Value=weight/32.2
  CG : Outport
  Inertia : Outport  Port=2
  mass : Outport  Port=3
  wires:
  cg/1 -> CG/1
  jy/1 -> Mux1/2
  jx/1 -> Mux1/1
  jz/1 -> Mux1/3
  jxz/1 -> Mux1/4
  Mux1/1 -> Inertia/1
  mass2/1 -> mass/1

== system Starfighter_6DoF_runsim_waypoint/Aircraft_Dynamics/Standard Atmosphere ==
  Position : Inport
  Constant : Constant  Value=rho
  Constant1 : Constant  Value=a
  Demux : Demux  Outputs=3
  Density : Fcn  Expr=2.3769e-3*(1 - 0.703e-5 * u[1])^4.14
  OATemp : Lookup  InputValues=[0 35000 60000]  Table=[519 390 390]  SaturateOnIntegerOverflow=on
  Speed of Sound : Fcn  Expr=sqrt(1.4*1716.3*u[1])
  Terminator{,1..3} (4 alike) : Terminator
  OAT : Outport
  rho : Outport  Port=2
  a : Outport  Port=3
  Hp : Outport  Port=4
  wires:
  OATemp/1 -> OAT/1, Speed of Sound/1
  Position/1 -> Demux/1
  Demux/1 -> Terminator/1
  Demux/2 -> Terminator1/1
  Demux/3 -> OATemp/1, Density/1, Hp/1
  Constant/1 -> rho/1
  Density/1 -> Terminator2/1
  Constant1/1 -> a/1
  Speed of Sound/1 -> Terminator3/1

== system Starfighter_6DoF_runsim_waypoint/Roll Control Add Pi Bound and Roll Saturation/pi Bound1 ==
  In : Inport
  2pi : Constant  Value=2*pi
  Math Function : Math  Operator=mod  SaturateOnIntegerOverflow=on
  Sum1 : Sum  Inputs=|+-  SaturateOnIntegerOverflow=on  InputSameDT=on  OutDataTypeStr=Inherit: Same as first input
  Sum2 : Sum  Inputs=|++  SaturateOnIntegerOverflow=on  InputSameDT=on  OutDataTypeStr=Inherit: Same as first input
  pi : Constant  Value=pi
  Out : Outport
  wires:
  Sum1/1 -> Out/1
  pi/1 -> Sum1/2, Sum2/2
  Sum2/1 -> Math Function/1
  In/1 -> Sum2/1
  2pi/1 -> Math Function/2
  Math Function/1 -> Sum1/1

== system Starfighter_6DoF_runsim_waypoint/Aircraft_Dynamics/Aerodynamics/Aero Forces and Moments ==
  dyn(q) : Inport
  CD : Inport  Port=2
  CY : Inport  Port=3
  CL : Inport  Port=4
  Wind Para : Inport  Port=5
  Croll : Inport  Port=6
  CM : Inport  Port=7
  CN : Inport  Port=8
  Aerodynamic Forces : Subsystem
  Aerodynamic Moments : Subsystem
  Faero : Outport
  Maero : Outport  Port=2
  wires:
  dyn(q)/1 -> Aerodynamic Moments/1(dyn(q)), Aerodynamic Forces/5(dyn(q))
  CD/1 -> Aerodynamic Forces/1(CD)
  CY/1 -> Aerodynamic Forces/2(CY)
  CL/1 -> Aerodynamic Forces/3(CL)
  Wind Para/1 -> Aerodynamic Forces/4(Wind Para)
  Croll/1 -> Aerodynamic Moments/2(Croll)
  CM/1 -> Aerodynamic Moments/3(CM)
  CN/1 -> Aerodynamic Moments/4(CN)
  Aerodynamic Forces/1(FaeroBody) -> Faero/1
  Aerodynamic Moments/1(Maero) -> Maero/1

== system Starfighter_6DoF_runsim_waypoint/Aircraft_Dynamics/Aerodynamics/CD ==
  Wind Parameters : Inport
  Controls : Inport  Port=2
  Mach No. : Inport  Port=3
     {,1..5} (6 alike) : Terminator
  Demux : Demux  Outputs=3
  Demux1 : Demux
  Sum : Sum  Inputs=+++  SaturateOnIntegerOverflow=on
  cda : Gain  Gain=cda  SaturateOnIntegerOverflow=on  OutDataTypeStr=Inherit: Same as input  ParamDataTypeStr=Inherit: Same as input
  cdde : Gain  Gain=cdde  SaturateOnIntegerOverflow=on  OutDataTypeStr=Inherit: Same as input  ParamDataTypeStr=Inherit: Same as input
  cdo : Constant  Value=cdo
  CD : Outport
  wires:
  Wind Parameters/1 -> Demux/1
  Sum/1 -> CD/1
  Controls/1 -> Demux1/1
  cda/1 -> Sum/2
  Mach No./1 -> "   1"/1
  cdo/1 -> Sum/1
  Demux/1 -> "   2"/1
  Demux/3 -> "   "/1
  Demux/2 -> cda/1
  cdde/1 -> Sum/3
  Demux1/1 -> cdde/1
  Demux1/2 -> "   3"/1
  Demux1/3 -> "   4"/1
  Demux1/4 -> "   5"/1

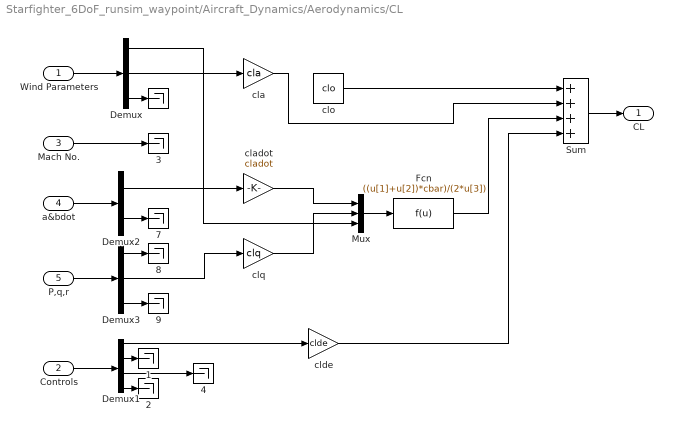
== system Starfighter_6DoF_runsim_waypoint/Aircraft_Dynamics/Aerodynamics/CL ==
  Wind Parameters : Inport
  Controls : Inport  Port=2
  Mach No. : Inport  Port=3
  a&bdot : Inport  Port=4
  P,q,r : Inport  Port=5
     {,1..4,7..9} (8 alike) : Terminator
  Demux : Demux  Outputs=3
  Demux1 : Demux
  Demux2 : Demux  Outputs=2
  Demux3 : Demux  Outputs=3
  Fcn : Fcn  Expr=((u[1]+u[2])*cbar)/(2*u[3])
  Mux : Mux  Inputs=3
  Sum : Sum  Inputs=++++  SaturateOnIntegerOverflow=on
  cla : Gain  Gain=cla  SaturateOnIntegerOverflow=on  OutDataTypeStr=Inherit: Same as input  ParamDataTypeStr=Inherit: Same as input
  cladot : Gain  Gain=cladot  SaturateOnIntegerOverflow=on  OutDataTypeStr=Inherit: Same as input  ParamDataTypeStr=Inherit: Same as input
  clde : Gain  Gain=clde  SaturateOnIntegerOverflow=on  OutDataTypeStr=Inherit: Same as input  ParamDataTypeStr=Inherit: Same as input
  clo : Constant  Value=clo
  clq : Gain  Gain=clq  SaturateOnIntegerOverflow=on  OutDataTypeStr=Inherit: Same as input  ParamDataTypeStr=Inherit: Same as input
  CL : Outport
  wires:
  Mux/1 -> Fcn/1
  Demux/1 -> Mux/3
  clo/1 -> Sum/1
  Demux2/2 -> "   7"/1
  Demux3/1 -> "   8"/1
  Demux3/3 -> "   9"/1
  Wind Parameters/1 -> Demux/1
  Sum/1 -> CL/1
  Controls/1 -> Demux1/1
  a&bdot/1 -> Demux2/1
  P,q,r/1 -> Demux3/1
  Demux/3 -> "   "/1
  Demux1/4 -> "   2"/1
  cla/1 -> Sum/2
  Demux2/1 -> cladot/1
  cladot/1 -> Mux/1
  Demux/2 -> cla/1
  clq/1 -> Mux/2
  Mach No./1 -> "   3"/1
  Demux3/2 -> clq/1
  Demux1/1 -> clde/1
  Demux1/2 -> "   1"/1
  Demux1/3 -> "   4"/1
  Fcn/1 -> Sum/3
  clde/1 -> Sum/4

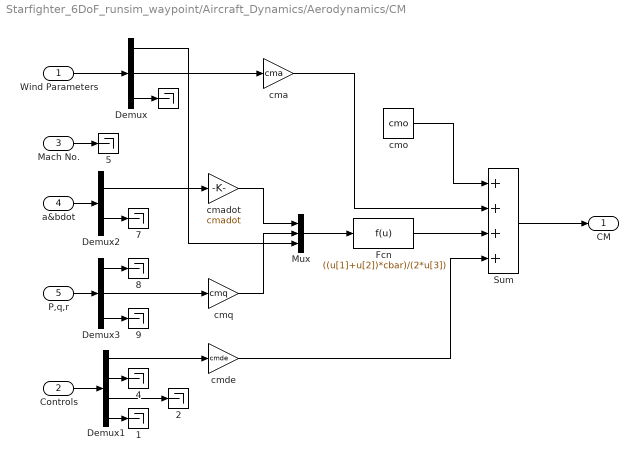
== system Starfighter_6DoF_runsim_waypoint/Aircraft_Dynamics/Aerodynamics/CM ==
  Wind Parameters : Inport
  Controls : Inport  Port=2
  Mach No. : Inport  Port=3
  a&bdot : Inport  Port=4
  P,q,r : Inport  Port=5
     {,1..2,4..5,7..9} (8 alike) : Terminator
  Demux : Demux  Outputs=3
  Demux1 : Demux
  Demux2 : Demux  Outputs=2
  Demux3 : Demux  Outputs=3
  Fcn : Fcn  Expr=((u[1]+u[2])*cbar)/(2*u[3])
  Mux : Mux  Inputs=3
  Sum : Sum  Inputs=++++  SaturateOnIntegerOverflow=on
  cma : Gain  Gain=cma  SaturateOnIntegerOverflow=on  OutDataTypeStr=Inherit: Same as input  ParamDataTypeStr=Inherit: Same as input
  cmadot : Gain  Gain=cmadot  SaturateOnIntegerOverflow=on  OutDataTypeStr=Inherit: Same as input  ParamDataTypeStr=Inherit: Same as input
  cmde : Gain  Gain=cmde  SaturateOnIntegerOverflow=on  OutDataTypeStr=Inherit: Same as input  ParamDataTypeStr=Inherit: Same as input
  cmo : Constant  Value=cmo
  cmq : Gain  Gain=cmq  SaturateOnIntegerOverflow=on  OutDataTypeStr=Inherit: Same as input  ParamDataTypeStr=Inherit: Same as input
  CM : Outport
  wires:
  Demux2/2 -> "   7"/1
  Demux3/1 -> "   8"/1
  Demux3/3 -> "   9"/1
  Wind Parameters/1 -> Demux/1
  Sum/1 -> CM/1
  Controls/1 -> Demux1/1
  a&bdot/1 -> Demux2/1
  P,q,r/1 -> Demux3/1
  Demux/3 -> "   "/1
  Demux1/4 -> "   1"/1
  Demux1/3 -> "   2"/1
  Demux/2 -> cma/1
  cmadot/1 -> Mux/1
  cmq/1 -> Mux/2
  Mux/1 -> Fcn/1
  Demux1/2 -> "   4"/1
  Mach No./1 -> "   5"/1
  Demux/1 -> Mux/3
  Demux1/1 -> cmde/1
  Demux2/1 -> cmadot/1
  Demux3/2 -> cmq/1
  Fcn/1 -> Sum/3
  cma/1 -> Sum/2
  cmde/1 -> Sum/4
  cmo/1 -> Sum/1

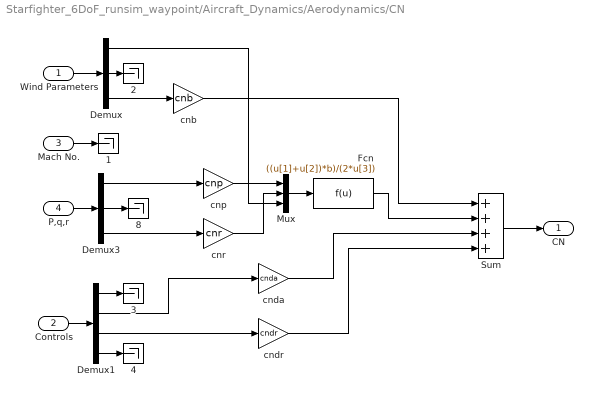
== system Starfighter_6DoF_runsim_waypoint/Aircraft_Dynamics/Aerodynamics/CN ==
  Wind Parameters : Inport
  Controls : Inport  Port=2
  Mach No. : Inport  Port=3
  P,q,r : Inport  Port=4
     {1..4,8} (5 alike) : Terminator
  Demux : Demux  Outputs=3
  Demux1 : Demux
  Demux3 : Demux  Outputs=3
  Fcn : Fcn  Expr=((u[1]+u[2])*b)/(2*u[3])
  Mux : Mux  Inputs=3
  Sum : Sum  Inputs=++++  SaturateOnIntegerOverflow=on
  cnb : Gain  Gain=cnb  SaturateOnIntegerOverflow=on  OutDataTypeStr=Inherit: Same as input  ParamDataTypeStr=Inherit: Same as input
  cnda : Gain  Gain=cnda  SaturateOnIntegerOverflow=on  OutDataTypeStr=Inherit: Same as input  ParamDataTypeStr=Inherit: Same as input
  cndr : Gain  Gain=cndr  SaturateOnIntegerOverflow=on  OutDataTypeStr=Inherit: Same as input  ParamDataTypeStr=Inherit: Same as input
  cnp : Gain  Gain=cnp  SaturateOnIntegerOverflow=on  OutDataTypeStr=Inherit: Same as input  ParamDataTypeStr=Inherit: Same as input
  cnr : Gain  Gain=cnr  SaturateOnIntegerOverflow=on  OutDataTypeStr=Inherit: Same as input  ParamDataTypeStr=Inherit: Same as input
  CN : Outport
  wires:
  Mux/1 -> Fcn/1
  Demux/2 -> "   2"/1
  Wind Parameters/1 -> Demux/1
  Sum/1 -> CN/1
  Controls/1 -> Demux1/1
  P,q,r/1 -> Demux3/1
  Demux3/2 -> "   8"/1
  cnb/1 -> Sum/1
  Mach No./1 -> "   1"/1
  Demux/3 -> cnb/1
  Demux/1 -> Mux/3
  Demux3/1 -> cnp/1
  cnp/1 -> Mux/1
  Demux3/3 -> cnr/1
  cnr/1 -> Mux/2
  Demux1/2 -> cnda/1
  Demux1/3 -> cndr/1
  Fcn/1 -> Sum/2
  cnda/1 -> Sum/3
  cndr/1 -> Sum/4
  Demux1/1 -> "   3"/1
  Demux1/4 -> "   4"/1

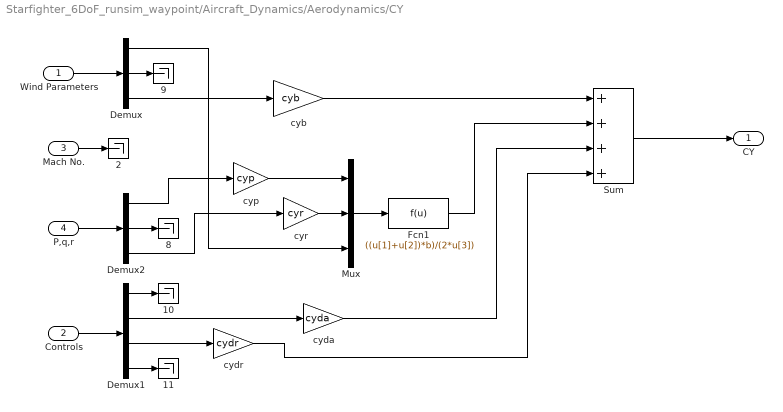
== system Starfighter_6DoF_runsim_waypoint/Aircraft_Dynamics/Aerodynamics/CY ==
  Wind Parameters : Inport
  Controls : Inport  Port=2
  Mach No. : Inport  Port=3
  P,q,r : Inport  Port=4
     {2,8..11} (5 alike) : Terminator
  Demux : Demux  Outputs=3
  Demux1 : Demux
  Demux2 : Demux  Outputs=3
  Fcn1 : Fcn  Expr=((u[1]+u[2])*b)/(2*u[3])
  Mux : Mux  Inputs=3
  Sum : Sum  Inputs=++++  SaturateOnIntegerOverflow=on
  cyb : Gain  Gain=cyb  SaturateOnIntegerOverflow=on  OutDataTypeStr=Inherit: Same as input  ParamDataTypeStr=Inherit: Same as input
  cyda : Gain  Gain=cyda  SaturateOnIntegerOverflow=on  OutDataTypeStr=Inherit: Same as input  ParamDataTypeStr=Inherit: Same as input
  cydr : Gain  Gain=cydr  SaturateOnIntegerOverflow=on  OutDataTypeStr=Inherit: Same as input  ParamDataTypeStr=Inherit: Same as input
  cyp : Gain  Gain=cyp  SaturateOnIntegerOverflow=on  OutDataTypeStr=Inherit: Same as input  ParamDataTypeStr=Inherit: Same as input
  cyr : Gain  Gain=cyr  SaturateOnIntegerOverflow=on  OutDataTypeStr=Inherit: Same as input  ParamDataTypeStr=Inherit: Same as input
  CY : Outport
  wires:
  Demux/2 -> "   9"/1
  Wind Parameters/1 -> Demux/1
  Sum/1 -> CY/1
  Controls/1 -> Demux1/1
  Demux/3 -> cyb/1
  Mach No./1 -> "   2"/1
  Demux1/3 -> cydr/1
  Demux1/1 -> "   10"/1
  Demux1/2 -> cyda/1
  Demux1/4 -> "   11"/1
  cyb/1 -> Sum/1
  Demux/1 -> Mux/3
  P,q,r/1 -> Demux2/1
  cydr/1 -> Sum/4
  cyda/1 -> Sum/3
  Mux/1 -> Fcn1/1
  Fcn1/1 -> Sum/2
  Demux2/2 -> "   8"/1
  Demux2/1 -> cyp/1
  Demux2/3 -> cyr/1
  cyp/1 -> Mux/1
  cyr/1 -> Mux/2

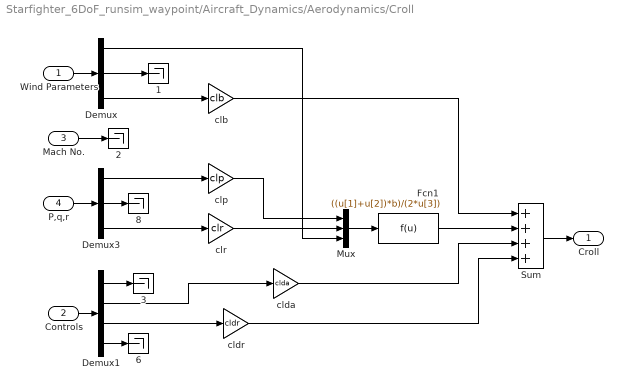
== system Starfighter_6DoF_runsim_waypoint/Aircraft_Dynamics/Aerodynamics/Croll ==
  Wind Parameters : Inport
  Controls : Inport  Port=2
  Mach No. : Inport  Port=3
  P,q,r : Inport  Port=4
     {1..3,6,8} (5 alike) : Terminator
  Demux : Demux  Outputs=3
  Demux1 : Demux
  Demux3 : Demux  Outputs=3
  Fcn1 : Fcn  Expr=((u[1]+u[2])*b)/(2*u[3])
  Mux : Mux  Inputs=3
  Sum : Sum  Inputs=++++  SaturateOnIntegerOverflow=on
  clb : Gain  Gain=clb  SaturateOnIntegerOverflow=on  OutDataTypeStr=Inherit: Same as input  ParamDataTypeStr=Inherit: Same as input
  clda : Gain  Gain=clda  SaturateOnIntegerOverflow=on  OutDataTypeStr=Inherit: Same as input  ParamDataTypeStr=Inherit: Same as input
  cldr : Gain  Gain=cldr  SaturateOnIntegerOverflow=on  OutDataTypeStr=Inherit: Same as input  ParamDataTypeStr=Inherit: Same as input
  clp : Gain  Gain=clp  SaturateOnIntegerOverflow=on  OutDataTypeStr=Inherit: Same as input  ParamDataTypeStr=Inherit: Same as input
  clr : Gain  Gain=clr  SaturateOnIntegerOverflow=on  OutDataTypeStr=Inherit: Same as input  ParamDataTypeStr=Inherit: Same as input
  Croll : Outport
  wires:
  Mux/1 -> Fcn1/1
  Demux/2 -> "   1"/1
  Wind Parameters/1 -> Demux/1
  Sum/1 -> Croll/1
  Controls/1 -> Demux1/1
  P,q,r/1 -> Demux3/1
  Demux3/2 -> "   8"/1
  Demux1/1 -> "   3"/1
  clp/1 -> Mux/1
  clb/1 -> Sum/1
  Demux/1 -> Mux/3
  Demux/3 -> clb/1
  Mach No./1 -> "   2"/1
  Demux3/1 -> clp/1
  Fcn1/1 -> Sum/2
  Demux3/3 -> clr/1
  clr/1 -> Mux/2
  Demux1/4 -> "   6"/1
  Demux1/2 -> clda/1
  Demux1/3 -> cldr/1
  clda/1 -> Sum/3
  cldr/1 -> Sum/4

== system Starfighter_6DoF_runsim_waypoint/Aircraft_Dynamics/Equations of motion numerical integration /Flat Earth Navigation ==
  note: 1  roll
      | 2  pitch
      | 3  yaw
      | 4 u
      | 5 v
      | 6 w
  Euler Angles : Inport
  Velocity : Inport  Port=2
  Alt : Integrator  InitialCondition=initalt
  Alttitude Dot : Fcn  Expr=u[4] * sin(u[2]) - u[5] * sin(u[1]) * cos(u[2]) - u[6] * cos(u[1]) * cos(u[2])
  Demux : Demux  Outputs=3
  Demux1 : Demux  Outputs=3
  East : Integrator  InitialCondition=initeast
  East Dot : Fcn  Expr=u[4] * cos(u[2])* sin(u[3]) + u[5] * (cos(u[1])*cos(u[3]) + sin(u[1])*sin(u[2])*sin(u[3])) + u[6] * (-sin(u[1])*cos(u[3])+cos(u[1])*sin(u[2])*sin(u[3]))
  Mux : Mux  Inputs=6
  Mux1 : Mux  Inputs=3
  North : Integrator  InitialCondition=initnorth
  North Dot : Fcn  Expr=u[4] * cos(u[2]) * cos(u[3]) + u[5]*(-cos(u[1])*sin(u[3])+sin(u[1])*sin(u[2])*sin(u[3]))+u[6]*(sin(u[1])*sin(u[3])+cos(u[1])*sin(u[2])*cos(u[3]))
  Position : Outport
  wires:
  Euler Angles/1 -> Demux/1
  Velocity/1 -> Demux1/1
  Demux/1 -> Mux/1
  Demux/2 -> Mux/2
  Demux/3 -> Mux/3
  Demux1/1 -> Mux/4
  Demux1/2 -> Mux/5
  Demux1/3 -> Mux/6
  Mux/1 -> East Dot/1, Alttitude Dot/1, North Dot/1
  East Dot/1 -> East/1
  North Dot/1 -> North/1
  Alttitude Dot/1 -> Alt/1
  East/1 -> Mux1/2
  North/1 -> Mux1/1
  Alt/1 -> Mux1/3
  Mux1/1 -> Position/1

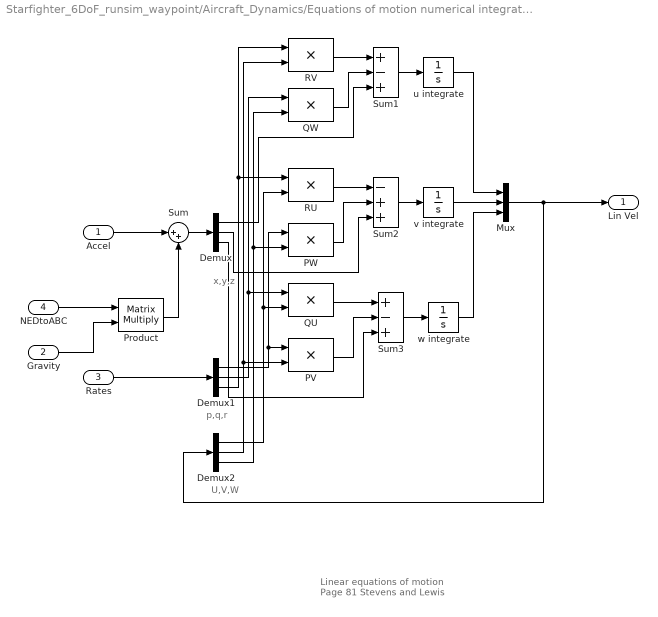
== system Starfighter_6DoF_runsim_waypoint/Aircraft_Dynamics/Equations of motion numerical integration /Force Equations ==
  note: U,V,W
  note: p,q,r
  note: x,y,z
  note: Linear equations of motion
      | Page 81 Stevens and Lewis
  Accel : Inport
  Gravity : Inport  Port=2
  Rates : Inport  Port=3
  NEDtoABC : Inport  Port=4
  Demux : Demux  Outputs=3
  Demux1 : Demux  Outputs=3
  Demux2 : Demux  Outputs=3
  Mux : Mux  Inputs=3
  PV : Product  SaturateOnIntegerOverflow=on  OutDataTypeStr=Inherit: Same as first input
  PW : Product  SaturateOnIntegerOverflow=on  OutDataTypeStr=Inherit: Same as first input
  Product : Product  Multiplication=Matrix(*)  SaturateOnIntegerOverflow=on  OutDataTypeStr=Inherit: Same as first input
  QU : Product  SaturateOnIntegerOverflow=on  OutDataTypeStr=Inherit: Same as first input
  QW : Product  SaturateOnIntegerOverflow=on  OutDataTypeStr=Inherit: Same as first input
  RU : Product  SaturateOnIntegerOverflow=on  OutDataTypeStr=Inherit: Same as first input
  RV : Product  SaturateOnIntegerOverflow=on  OutDataTypeStr=Inherit: Same as first input
  Sum : Sum  Inputs=|++  SaturateOnIntegerOverflow=on
  Sum1 : Sum  Inputs=+-+  SaturateOnIntegerOverflow=on
  Sum2 : Sum  Inputs=-++  SaturateOnIntegerOverflow=on
  Sum3 : Sum  Inputs=+-+  SaturateOnIntegerOverflow=on
  u integrate : Integrator  InitialCondition=initu
  v integrate : Integrator  InitialCondition=initv
  w integrate : Integrator  InitialCondition=initw
  Lin Vel : Outport
  wires:
  Sum/1 -> Demux/1
  Accel/1 -> Sum/1
  Rates/1 -> Demux1/1
  Mux/1 -> Demux2/1, Lin Vel/1
  Demux1/3 -> RV/1, RU/1
  Demux2/2 -> RV/2, PV/2
  RV/1 -> Sum1/1
  Demux1/2 -> QW/1, QU/1
  Demux2/3 -> QW/2, PW/2
  QW/1 -> Sum1/2
  Demux/1 -> Sum1/3
  Demux2/1 -> RU/2, QU/2
  RU/1 -> Sum2/1
  Demux1/1 -> PV/1, PW/1
  PW/1 -> Sum2/2
  Demux/2 -> Sum2/3
  QU/1 -> Sum3/1
  PV/1 -> Sum3/2
  Demux/3 -> Sum3/3
  Gravity/1 -> Product/2
  NEDtoABC/1 -> Product/1
  Product/1 -> Sum/2
  Sum1/1 -> u integrate/1
  Sum2/1 -> v integrate/1
  Sum3/1 -> w integrate/1
  u integrate/1 -> Mux/1
  v integrate/1 -> Mux/2
  w integrate/1 -> Mux/3

== system Starfighter_6DoF_runsim_waypoint/Aircraft_Dynamics/Equations of motion numerical integration /Gravity Model ==
  Constant : Constant  Value=0
  Constant1 : Constant  Value=32.2
  Mux : Mux  Inputs=3
  Gravity : Outport
  wires:
  Constant/1 -> Mux/1, Mux/2
  Constant1/1 -> Mux/3
  Mux/1 -> Gravity/1

== system Starfighter_6DoF_runsim_waypoint/Aircraft_Dynamics/Equations of motion numerical integration /Inert-body ==
  Euler : Inport
  11 : Fcn  Expr=cos(u[2])*cos(u[3])
  12 : Fcn  Expr=-cos(u[1])*sin(u[3])+sin(u[1])*sin(u[2])*cos(u[3])
  13 : Fcn  Expr=sin(u[1])*sin(u[3])+cos(u[1])*sin(u[2])*cos(u[3])
  21 : Fcn  Expr=cos(u[2])*sin(u[3])
  22 : Fcn  Expr=cos(u[1])*cos(u[3]) + sin(u[1])*sin(u[2])*sin(u[3])
  23 : Fcn  Expr=-sin(u[1])*cos(u[3])+cos(u[1])*sin(u[2])*sin(u[3])
  31 : Fcn  Expr=-sin(u[2])
  32 : Fcn  Expr=sin(u[1]) * cos(u[2])
  33 : Fcn  Expr=cos(u[1])*cos(u[2])
  Matrix Concatenation : Concatenate  NumInputs=3  Mode=Multidimensional array
  Matrix Concatenation1 : Concatenate  NumInputs=3  Mode=Multidimensional array
  Matrix Concatenation2 : Concatenate  NumInputs=3  Mode=Multidimensional array
  Matrix Concatenation3 : Concatenate  NumInputs=3  Mode=Multidimensional array  ConcatenateDimension=2
  NEDtoBC : Outport
  wires:
  Euler/1 -> 11/1, 12/1, 13/1, 21/1, 22/1, 23/1, 31/1, 33/1, 32/1
  12/1 -> Matrix Concatenation/2
  11/1 -> Matrix Concatenation/1
  13/1 -> Matrix Concatenation/3
  22/1 -> Matrix Concatenation1/2
  21/1 -> Matrix Concatenation1/1
  23/1 -> Matrix Concatenation1/3
  32/1 -> Matrix Concatenation2/2
  31/1 -> Matrix Concatenation2/1
  33/1 -> Matrix Concatenation2/3
  Matrix Concatenation1/1 -> Matrix Concatenation3/2
  Matrix Concatenation/1 -> Matrix Concatenation3/1
  Matrix Concatenation2/1 -> Matrix Concatenation3/3
  Matrix Concatenation3/1 -> NEDtoBC/1

== system Starfighter_6DoF_runsim_waypoint/Aircraft_Dynamics/Equations of motion numerical integration /Kinematic Equiations ==
  note: 1  p
      | 2  q
      | 3  r
      | 4  roll
      | 5 pitch
      | 6 yaw
  Rates : Inport
  Demux : Demux  Outputs=3
  Demux1 : Demux  Outputs=3
  Demux2 : Demux  Outputs=3
  Mux : Mux  Inputs=6
  Mux1 : Mux  Inputs=3
  Mux2 : Mux  Inputs=3
  Yaw rate : Fcn  Expr=(u[2] * sin(u[4]) + u[3] * cos(u[4]))/cos(u[5])
  pi Bound : Subsystem  mask(pi bound){}
      mask help: Bounds the input angle to [-pi, pi]. When -pi bound is exceeded the output wraps back to pi; when the pi bound is exceeded the output wraps back to -pi.
      mask Help:
      | Bounds the input angle to [-pi, pi]. When -pi bound is exceeded the output wraps back to pi; when the pi bound is exceeded the output wraps back to -pi.
      | <P><B>Input:</B> any angle in radians, from -Inf to Inf;</P>
      | <P><B>Output:</B> an angle in radians between -pi and pi.</P>
  pi Bound1 : Subsystem  mask(pi bound){}
      mask help: Bounds the input angle to [-pi, pi]. When -pi bound is exceeded the output wraps back to pi; when the pi bound is exceeded the output wraps back to -pi.
      mask Help:
      | Bounds the input angle to [-pi, pi]. When -pi bound is exceeded the output wraps back to pi; when the pi bound is exceeded the output wraps back to -pi.
      | <P><B>Input:</B> any angle in radians, from -Inf to Inf;</P>
      | <P><B>Output:</B> an angle in radians between -pi and pi.</P>
  pitch : Integrator  InitialCondition=initpitch
  pitch rate : Fcn  Expr=u[2] *cos(u[4]) - u[3] * sin(u[4])
  roll : Integrator  InitialCondition=initroll
  roll rate : Fcn  Expr=u[1] + tan(u[5])*(u[2]*sin(u[4])+u[3]*cos(u[4]))
  yaw : Integrator  InitialCondition=inityaw
  Euler angles : Outport
  wires:
  Rates/1 -> Demux/1
  Demux/2 -> Mux/2
  Demux/3 -> Mux/3
  Demux1/1 -> Mux/4
  Demux1/2 -> Mux/5
  Demux1/3 -> Mux/6
  Demux/1 -> Mux/1
  Mux/1 -> roll rate/1, Yaw rate/1, pitch rate/1
  Demux2/2 -> pi Bound/1(In)
  Demux2/1 -> pi Bound1/1(In)
  Mux2/1 -> Euler angles/1
  pi Bound/1(Out) -> Mux2/2
  pi Bound1/1(Out) -> Mux2/1
  Demux2/3 -> Mux2/3
  pitch rate/1 -> pitch/1
  roll rate/1 -> roll/1
  Yaw rate/1 -> yaw/1
  roll/1 -> Mux1/1
  pitch/1 -> Mux1/2
  yaw/1 -> Mux1/3
  Mux1/1 -> Demux2/1, Demux1/1

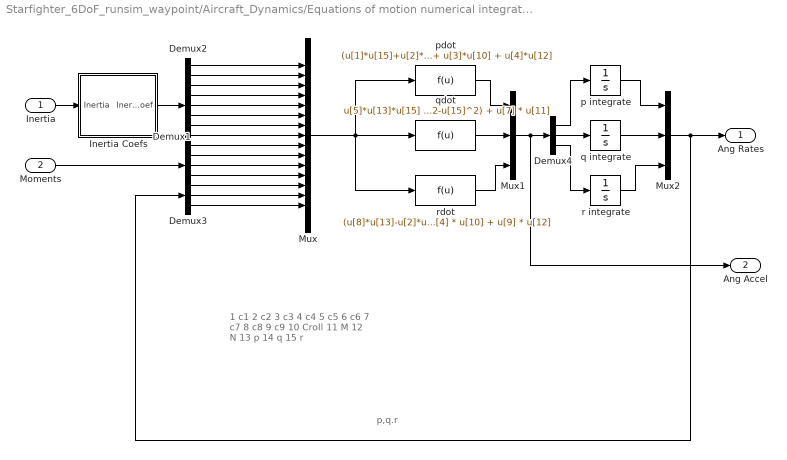
== system Starfighter_6DoF_runsim_waypoint/Aircraft_Dynamics/Equations of motion numerical integration /Moment Equations ==
  note: 1   c1
      | 2   c2
      | 3   c3
      | 4  c4
      | 5  c5
      | 6  c6
      | 7  c7
      | 8  c8
      | 9  c9
      | 10 Croll
      | 11  M
      | 12  N
      | 13  p
      | 14  q
      | 15  r
  note: p,q.r
  Inertia : Inport
  Moments : Inport  Port=2
  Demux1 : Demux  Outputs=3
  Demux2 : Demux  Outputs=9
  Demux3 : Demux  Outputs=3
  Demux4 : Demux  Outputs=3
  Inertia Coefs : Subsystem
  Mux : Mux  Inputs=15
  Mux1 : Mux  Inputs=3
  Mux2 : Mux  Inputs=3
  p integrate : Integrator  InitialCondition=initp
  pdot : Fcn  Expr=(u[1]*u[15]+u[2]*u[13])*u[14] + u[3]*u[10] + u[4]*u[12]
  q integrate : Integrator  InitialCondition=initq
  qdot : Fcn  Expr=u[5]*u[13]*u[15] - u[6]*(u[13]^2-u[15]^2) + u[7] * u[11]
  r integrate : Integrator  InitialCondition=initr
  rdot : Fcn  Expr=(u[8]*u[13]-u[2]*u[15]) * u[14] + u[4] * u[10] + u[9] * u[12]
  Ang Rates : Outport
  Ang Accel : Outport  Port=2
  wires:
  Inertia/1 -> Inertia Coefs/1(Inertia)
  Moments/1 -> Demux1/1
  Inertia Coefs/1(Iner Coef) -> Demux2/1
  Demux2/1 -> Mux/1
  Demux2/2 -> Mux/2
  Demux2/3 -> Mux/3
  Demux2/4 -> Mux/4
  Demux2/5 -> Mux/5
  Demux2/6 -> Mux/6
  Demux2/7 -> Mux/7
  Demux2/8 -> Mux/8
  Demux2/9 -> Mux/9
  Demux1/1 -> Mux/10
  Demux1/2 -> Mux/11
  Demux1/3 -> Mux/12
  Demux3/1 -> Mux/13
  Demux3/2 -> Mux/14
  Demux3/3 -> Mux/15
  Mux/1 -> pdot/1, qdot/1, rdot/1
  qdot/1 -> Mux1/2
  pdot/1 -> Mux1/1
  rdot/1 -> Mux1/3
  Mux1/1 -> Ang Accel/1, Demux4/1
  Demux4/1 -> p integrate/1
  Demux4/2 -> q integrate/1
  Demux4/3 -> r integrate/1
  Mux2/1 -> Ang Rates/1, Demux3/1
  p integrate/1 -> Mux2/1
  q integrate/1 -> Mux2/2
  r integrate/1 -> Mux2/3

== system Starfighter_6DoF_runsim_waypoint/Aircraft_Dynamics/Linear Acc and Moments/Cross Prod Moment due Leng ==
  Vec 1 : Inport
  Vec 2 : Inport  Port=2
  Check prob not zero : Constant  Value=0
  Demux : Demux  Outputs=3
  J axis : Fcn  Expr=u[4]*u[3] - u[6]*u[1]
  Mux : Mux  Inputs=6
  Mux1 : Mux  Inputs=3
  i axis : Fcn  Expr=u[6]*u[2] - u[5]*u[3]
  k axis : Fcn  Expr=u[5]*u[1] - u[4]*u[2]
  X Prod : Outport
  wires:
  Vec 2/1 -> Mux/4
  Vec 1/1 -> Demux/1
  Demux/1 -> Mux/1
  Check prob not zero/1 -> Mux/5, Mux/6
  Demux/3 -> Mux/3
  Demux/2 -> Mux/2
  Mux/1 -> i axis/1, J axis/1, k axis/1
  J axis/1 -> Mux1/2
  i axis/1 -> Mux1/1
  k axis/1 -> Mux1/3
  Mux1/1 -> X Prod/1

== system Starfighter_6DoF_runsim_waypoint/Aircraft_Dynamics/Linear Acc and Moments/Cross Prod Moment due to Aero ==
  Vec 1 : Inport
  Vec 2 : Inport  Port=2
  Demux : Demux  Outputs=3
  Demux1 : Demux  Outputs=3
  J axis : Fcn  Expr=u[4]*u[3] - u[6]*u[1]
  Mux : Mux  Inputs=6
  Mux1 : Mux  Inputs=3
  i axis : Fcn  Expr=u[6]*u[2] - u[5]*u[3]
  k axis : Fcn  Expr=u[5]*u[1] - u[4]*u[2]
  X Prod : Outport
  wires:
  Vec 2/1 -> Demux1/1
  Vec 1/1 -> Demux/1
  Demux/1 -> Mux/1
  Demux1/3 -> Mux/6
  Demux1/2 -> Mux/5
  Demux1/1 -> Mux/4
  Demux/3 -> Mux/3
  Demux/2 -> Mux/2
  Mux/1 -> i axis/1, J axis/1, k axis/1
  J axis/1 -> Mux1/2
  i axis/1 -> Mux1/1
  k axis/1 -> Mux1/3
  Mux1/1 -> X Prod/1
